simulink model "inverseKinematicsRobotics"  (R2023a)
settings: Solver=VariableStepAuto  StartTime=0.0  StopTime=10.0  RelTol=1e-3
libraries: simulink_extras x2
settings Model: Creator=Dina  LastModifiedBy=Dina

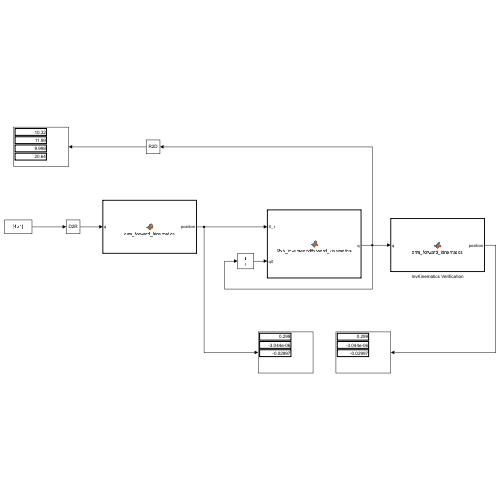
[thumbnail: Simulink's stored preview of the top-level diagram]
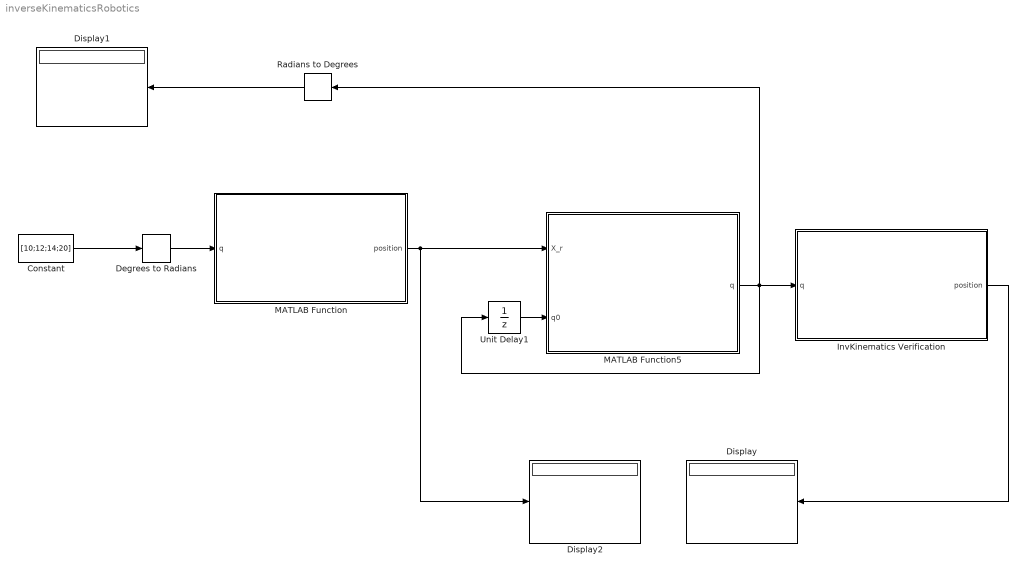
== system inverseKinematicsRobotics ==
  Constant : Constant  Value=[10;12;14;20]
  Degrees to Radians : simulink_extras/Transformations/Degrees to Radians
  Display : Display
  Display1 : Display
  Display2 : Display
  InvKinematics Verification : MATLAB Function  TreatAsAtomicUnit=on
  MATLAB Function : MATLAB Function  TreatAsAtomicUnit=on
  MATLAB Function5 : MATLAB Function  TreatAsAtomicUnit=on
  Radians to Degrees : simulink_extras/Transformations/Radians to Degrees
  Unit Delay1 : UnitDelay  InitialCondition=deg2rad([9;10;10;5])  SampleTime=-1  HasFrameUpgradeWarning=on
  wires:
  MATLAB Function5/1(q) -> Radians to Degrees/1, Unit Delay1/1, InvKinematics Verification/1(q)
  Unit Delay1/1 -> MATLAB Function5/2(q0)
  Constant/1 -> Degrees to Radians/1
  MATLAB Function/1(position) -> MATLAB Function5/1(X_r), Display2/1
  InvKinematics Verification/1(position) -> Display/1
  Radians to Degrees/1 -> Display1/1
  Degrees to Radians/1 -> MATLAB Function/1(q)

== matlab function inverseKinematicsRobotics/MATLAB Function5 ==
  data: X_r input; q output; q0 input
function q   = Rob_inverseandforward_kinematics(X_r,q0)
    l1 = 0.0288811487749;%old: 0.0291
    l2 = 0.02659997;%old: 0.04406
    l3 = 0.12240002;%old: 0.10416
    l4 = 0.15;%old: 0.15444
    x=0;
    y=0;
    z=0;
    J = zeros(3,4);
    %Calculate the inverse Jacobian matrix
    
    q = q0 ;
    maxError = 10^-8;
    error = inf;
     % 
     while error > maxError
            
            q1 = q(1,1);
            q2 = q(2,1);
            q3 = q(3,1);
            q4 = q(4,1);
            
          
    
    X = [l4*cos((pi*q1)/180)*sin((pi*(q2 - 90))/180)*sin((pi*(q4 - 90))/180)-l4*cos((pi*(q4 - 90))/180)*(sin((pi*q1)/180)*sin((pi*(q3 - 90))/180)-cos((pi*q1)/180)*cos((pi*(q2 - 90))/180)*cos((pi*(q3 - 90))/180))-cos((pi*q1)/180)*sin((pi*(q2 - 90))/180)*(l2 + l3);
        l4*cos((pi*(q4 - 90))/180)*(cos((pi*q1)/180)*sin((pi*(q3 - 90))/180)+sin((pi*q1)/180)*cos((pi*(q2 - 90))/180)*cos((pi*(q3 - 90))/180))-sin((pi*q1)/180)*sin((pi*(q2 - 90))/180)*(l2 + l3)+l4*sin((pi*q1)/180)*sin((pi*(q2 - 90))/180)*sin((pi*(q4 - 90))/180);
        l4*cos((pi*(q2 - 90))/180)*sin((pi*(q4 - 90))/180)-cos((pi*(q2 - 90))/180)*(l2 + l3)-l1-l4*cos((pi*(q3 - 90))/180)*cos((pi*(q4 - 90))/180)*sin((pi*(q2 - 90))/180)];
 
    x = X(1,1);
    y = X(2,1);
    z = X(3,1);
           
    
            x_current = [x;y;z];
             
           
            % if error < maxError
            %     break;
            % end
     
            Jac= [(l4*pi*sin((pi*q4)/180)*(cos((pi*q1)/180)*cos((pi*q3)/180)-sin((pi*q1)/180)*sin((pi*q2)/180)*sin((pi*q3)/180)))/180 - (pi*cos((pi*q2)/180)*sin((pi*q1)/180)*(l2 + l3))/180 - (l4*pi*cos((pi*q2)/180)*cos((pi*q4)/180)*sin((pi*q1)/180))/180,                          -(pi*cos((pi*q1)/180)*(l2*sin((pi*q2)/180) + l3*sin((pi*q2)/180) + l4*cos((pi*q4)/180)*sin((pi*q2)/180) - l4*cos((pi*q2)/180)*sin((pi*q3)/180)*sin((pi*q4)/180)))/180, -(l4*pi*sin((pi*q4)/180)*(sin((pi*q1)/180)*sin((pi*q3)/180) - cos((pi*q1)/180)*cos((pi*q3)/180)*sin((pi*q2)/180)))/180,   (l4*pi*cos((pi*q4)/180)*(cos((pi*q3)/180)*sin((pi*q1)/180) + cos((pi*q1)/180)*sin((pi*q2)/180)*sin((pi*q3)/180)))/180 - (l4*pi*cos((pi*q1)/180)*cos((pi*q2)/180)*sin((pi*q4)/180))/180;
                 (l4*pi*sin((pi*q4)/180)*(cos((pi*q3)/180)*sin((pi*q1)/180)+ cos((pi*q1)/180)*sin((pi*q2)/180)*sin((pi*q3)/180)))/180 + (pi*cos((pi*q1)/180)*cos((pi*q2)/180)*(l2 + l3))/180 + (l4*pi*cos((pi*q1)/180)*cos((pi*q2)/180)*cos((pi*q4)/180))/180,                          -(pi*sin((pi*q1)/180)*(l2*sin((pi*q2)/180) + l3*sin((pi*q2)/180) + l4*cos((pi*q4)/180)*sin((pi*q2)/180) - l4*cos((pi*q2)/180)*sin((pi*q3)/180)*sin((pi*q4)/180)))/180,  (l4*pi*sin((pi*q4)/180)*(cos((pi*q1)/180)*sin((pi*q3)/180) + cos((pi*q3)/180)*sin((pi*q1)/180)*sin((pi*q2)/180)))/180, - (l4*pi*cos((pi*q4)/180)*(cos((pi*q1)/180)*cos((pi*q3)/180) - sin((pi*q1)/180)*sin((pi*q2)/180)*sin((pi*q3)/180)))/180 - (l4*pi*cos((pi*q2)/180)*sin((pi*q1)/180)*sin((pi*q4)/180))/180;
                                                                                                                                                                                                                                                      0, (pi*sin((pi*(q2 - 90))/180)*(l2 + l3))/180 - (l4*pi*sin((pi*(q2 - 90))/180)*sin((pi*(q4 - 90))/180))/180 - (l4*pi*cos((pi*(q2 - 90))/180)*cos((pi*(q3 - 90))/180)*cos((pi*(q4 - 90))/180))/180,                                                         (l4*pi*cos((pi*q2)/180)*cos((pi*q3)/180)*sin((pi*q4)/180))/180,                                                                           (l4*pi*sin((pi*q2)/180)*sin((pi*q4)/180))/180 + (l4*pi*cos((pi*q2)/180)*cos((pi*q4)/180)*sin((pi*q3)/180))/180;
                                                                                                                                                                                                                                                            0,                                                                                                                                                                        sin((pi*(q2 - 90))/180),                                                                                     -cos((pi*q3)/180)*sin((pi*q2)/180),                                                                                                                                                       -cos((pi*q3)/180)*sin((pi*q2)/180);
                                                                                                                                                                                                                                                      0,                                                                                                                                                                       -cos((pi*(q2 - 90))/180),                                                                                      cos((pi*q2)/180)*cos((pi*q3)/180),                                                                                                                                                        cos((pi*q2)/180)*cos((pi*q3)/180);
                                                                                                                                                                                                                                                       1,                                                                                                                                                                                              0,                                                                                               -cos((pi*(q3 - 90))/180),                                                                                                                                                                 -cos((pi*(q3 - 90))/180)]
            J = Jac(1:3,:);  
            fakeJ =pinv(J);
            x_error =  x_current-X_r;
            q = (double(q - fakeJ* x_error));
            % q=wrapToPi(q)
            error = norm(x_error);
          
        
        end

== matlab function inverseKinematicsRobotics/MATLAB Function ==
  data: q input; position output
function position  = arm_forward_kinematics(q)
    q1=q(1);
    q2=q(2);
    q3=q(3);
    q4=q(4);
    l1 = 0.02888114877;
    l2 = 0.0265999;
    l3 = 0.1224;
    l4 = 0.15;
    X = [l4*cos((pi*q1)/180)*sin((pi*(q2 - 90))/180)*sin((pi*(q4 - 90))/180) - l4*cos((pi*(q4 - 90))/180)*(sin((pi*q1)/180)*sin((pi*(q3 - 90))/180) - cos((pi*q1)/180)*cos((pi*(q2 - 90))/180)*cos((pi*(q3 - 90))/180)) - cos((pi*q1)/180)*sin((pi*(q2 - 90))/180)*(l2 + l3);
l4*cos((pi*(q4 - 90))/180)*(cos((pi*q1)/180)*sin((pi*(q3 - 90))/180) + sin((pi*q1)/180)*cos((pi*(q2 - 90))/180)*cos((pi*(q3 - 90))/180)) - sin((pi*q1)/180)*sin((pi*(q2 - 90))/180)*(l2 + l3) + l4*sin((pi*q1)/180)*sin((pi*(q2 - 90))/180)*sin((pi*(q4 - 90))/180);
                                                                                           l4*cos((pi*(q2 - 90))/180)*sin((pi*(q4 - 90))/180) - cos((pi*(q2 - 90))/180)*(l2 + l3) - l1 - l4*cos((pi*(q3 - 90))/180)*cos((pi*(q4 - 90))/180)*sin((pi*(q2 - 90))/180)]
 
    x = X(1,1);
    y = X(2,1);
    z = X(3,1);
    position=[x;y;z];

== matlab function inverseKinematicsRobotics/InvKinematics Verification ==
  data: q input; position output
function position  = arm_forward_kinematics(q)
    q1=q(1);
    q2=q(2);
    q3=q(3);
    q4=q(4);
    l1 = 0.02888114877;
    l2 = 0.0265999;
    l3 = 0.1224;
    l4 = 0.15;
    X = [l4*cos((pi*q1)/180)*sin((pi*(q2 - 90))/180)*sin((pi*(q4 - 90))/180) - l4*cos((pi*(q4 - 90))/180)*(sin((pi*q1)/180)*sin((pi*(q3 - 90))/180) - cos((pi*q1)/180)*cos((pi*(q2 - 90))/180)*cos((pi*(q3 - 90))/180)) - cos((pi*q1)/180)*sin((pi*(q2 - 90))/180)*(l2 + l3);
l4*cos((pi*(q4 - 90))/180)*(cos((pi*q1)/180)*sin((pi*(q3 - 90))/180) + sin((pi*q1)/180)*cos((pi*(q2 - 90))/180)*cos((pi*(q3 - 90))/180)) - sin((pi*q1)/180)*sin((pi*(q2 - 90))/180)*(l2 + l3) + l4*sin((pi*q1)/180)*sin((pi*(q2 - 90))/180)*sin((pi*(q4 - 90))/180);
                                                                                           l4*cos((pi*(q2 - 90))/180)*sin((pi*(q4 - 90))/180) - cos((pi*(q2 - 90))/180)*(l2 + l3) - l1 - l4*cos((pi*(q3 - 90))/180)*cos((pi*(q4 - 90))/180)*sin((pi*(q2 - 90))/180)]
 
    x = X(1,1);
    y = X(2,1);
    z = X(3,1);
    position=[x;y;z];
